simulink model "ee_converter_dcdc_llc"  (R2019b)
settings: Solver=VariableStepAuto  StartTime=0.0  StopTime=2e-3  RelTol=1e-3  AbsTol=1e-3  EnableMultiTasking=on
PreLoadFcn:
  | Vbus_nominal = 450;
  | Vbus_ripple = 10;
  | busRippleFrequency = 100;
  | Vout_nominal = 54;
  | Pout = 100;
  | Cr = 1.5e-8;
  | Lr = 2e-4;
  | Lm_theory = 2.5e-3;
  | n = 4.3;
  | transformerCoupling = 0.99;
  | Cout = 3e-5;
  | tdead = 3e-7;
  | fswfinal = [68.7 93.7]*1e3;
  | Vf = 0.6;
  | 
  | switchType = 1;
StopFcn:
  | ee_addSimlogTimeStamp(bdroot)
undefined symbols (not defined in the file or in its folder): diff
libraries: ee_lib x12, fl_lib x10, nesl_utility x6, simulink x4
(part 1 of 2)
CloseFcn:
  | try,close(h1_ee_converter_dcdc_llc),end
  | clear h1_ee_converter_dcdc_llc
  | try,close(h2_ee_converter_dcdc_llc),end
  | clear h2_ee_converter_dcdc_llc
  | try,close(h3_ee_converter_dcdc_llc),end
  | clear h3_ee_converter_dcdc_llc
  | try,close(h4_ee_converter_dcdc_llc),end
  | clear h4_ee_converter_dcdc_llc
  | try,close(h5_ee_converter_dcdc_llc),end
  | clear h5_ee_converter_dcdc_llc
  | 
  | clear simlog_ee_converter_dcdc_llc
  | clear logsout_ee_converter_dcdc_llc
  | clear simlogs_ee_converter_dcdc_llc
  | clear logsouts_ee_converter_dcdc_llc
  | 
  | clear Cout Cr G Gmax Gmax_factor Gmin Gnom Gnorm Gplot Iout Lm Lm_theory Lr Lr_theory Pout Q Qmaxfinal Qminfinal Qnomfinal Qplot Qrange Re Remax Remin Renom Vbus Vbus_nominal Vbus_ripple Vf Vout Vout_nominal Vout_ripple Zr busRippleFrequency ff ffinal fn fplot frange fsw fswfinal ii io lambda leg minLoad n nexact numCurves numPts qq showplots simlog_fctrl switchType tdead temp_ivar temp_variant tout transformerCoupling vi vo
Description:
  | DC-DC LLC Converter
settings Model: Creator=The MathWorks, Inc.  LastModifiedBy=sheldon
settings SolverCC: AutoScaleAbsTol=off  MaxConsecutiveMinStep=5
settings DataIOCC: LimitDataPoints=on  MaxDataPoints=400000  ReturnWorkspaceOutputs=off  SignalLoggingName=logsout_ee_converter_dcdc_llc
settings DebuggingCC: ArithmeticOperatorsInVariantConditions=warning
settings SFSimCC: SimUseLocalCustomCode=off  CustomCodeUndefinedFunction=UseInterfaceOnly
settings RTWCC: RTWUseLocalCustomCode=off
settings CodeAppCC: StateflowObjectComments=on
settings GRTTargetCC: TargetLangStandard=C89/C90 (ANSI)
settings ConfigComp: CovMetricSettings=dw  CovHtmlReporting=on  CovSaveCumulativeToWorkspaceVar=on  CovSaveSingleToWorkspaceVar=on  CovShowResultsExplorer=off  CovExternalEMLEnable=off
settings SimscapeCC: SimscapeLogType=all  SimscapeLogSimulationStatistics=on  SimscapeLogName=simlog_ee_converter_dcdc_llc  SimscapeLogDataHistory=400000

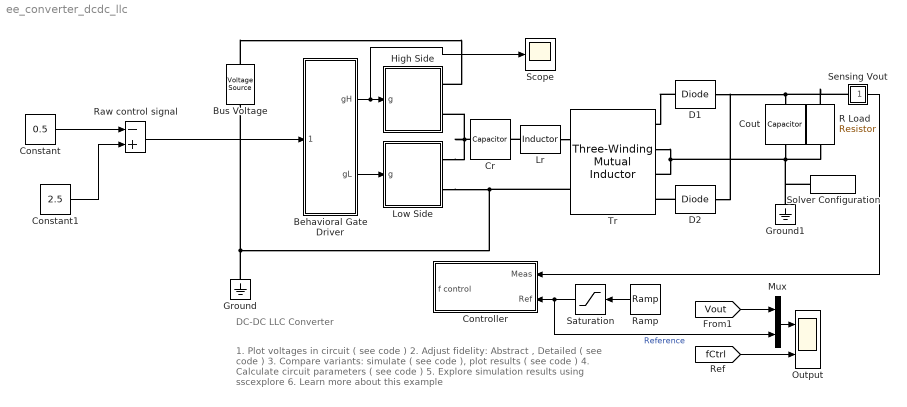
== system ee_converter_dcdc_llc ==
  note: DC-DC LLC Converter
  note: 1. Plot voltages in circuit ( see code )
      | 2. Adjust fidelity: Abstract , Detailed ( see code )
      | 3. Compare variants: simulate ( see code ), plot results ( see code )
      | 4. Calculate circuit parameters ( see code )
      | 5. Explore simulation results using sscexplore
      | 6. Learn more about this example
  Behavioral Gate Driver : Subsystem
  Bus Voltage : ee_lib/Sources/Voltage Source  dc_voltage=Vbus_nominal V  ac_voltage=Vbus_ripple V  ac_shift=0 deg  ac_frequency=busRippleFrequency Hz  noise_mode=0  PSD=0 V^2/Hz  repeatability=1  auto_seed=3499211588  user_seed=0  sample_time=0.001 s  i_specify=off  i_priority=None  i=0 A  i_nominal_specify=off  i_nominal_unit=A  i_nominal_value=1  v_specify=off  v_priority=None  v=0 V  v_nominal_specify=off  v_nominal_unit=V  v_nominal_value=1
      settings: SourceProductName=Simscape Electrical
  Constant : Constant  Value=0.5
  Constant1 : Constant  Value=2.5
  Controller : Subsystem
  Cout : ee_lib/Passive/Capacitor  cap_option=0  c=Cout F  Cvec=[ 1e-5 1e-6 ] F  Vvec=[ 0 10 ] V  CV_table_symmetry=1  f_vec=[1, 10] kHz  DFext_vec=[.8, 1.2]  C_tol=5  enable_C_tol=0  tol_distribution=1  nSigma=4  r=1e-6 Ohm  g=0 1/Ohm  averaging_period=0 s  enable_operating_limits=0  operating_limit_action=2  max_working_voltage_range=[ -25 25 ] V  power_rating=1 W  enable_faults=0  fault_action=1  Cscale_faulted=100  R_faulted=0.001 Ohm  G_faulted=0 1/Ohm  tau_fault=0.001 s  enable_temporal_fault=0  t_fault=1 s  enable_behavioral_fault=0  max_permissible_voltage_range=[ -100 100 ] V  t_fail_on_voltage=1 s  i_specify=off  i_priority=None  i=0 A  i_nominal_specify=off  i_nominal_unit=A  i_nominal_value=1  v_specify=off  v_priority=None  v=0 V  v_nominal_specify=off  v_nominal_unit=V  v_nominal_value=1  vc_specify=on  vc_priority=High  vc=0 V  vc_nominal_specify=off  vc_nominal_unit=V  vc_nominal_value=1
      settings: SourceProductName=Simscape Electrical
  Cr : ee_lib/Passive/Capacitor  cap_option=0  c=Cr F  Cvec=[ 1e-5 1e-6 ] F  Vvec=[ 0 10 ] V  CV_table_symmetry=1  f_vec=[1, 10] kHz  DFext_vec=[.8, 1.2]  C_tol=5  enable_C_tol=0  tol_distribution=1  nSigma=4  r=1e-6 Ohm  g=1e-6 1/Ohm  averaging_period=0 s  enable_operating_limits=0  operating_limit_action=2  max_working_voltage_range=[ -25 25 ] V  power_rating=1 W  enable_faults=0  fault_action=1  Cscale_faulted=100  R_faulted=0.001 Ohm  G_faulted=0 1/Ohm  tau_fault=0.001 s  enable_temporal_fault=0  t_fault=1 s  enable_behavioral_fault=0  max_permissible_voltage_range=[ -100 100 ] V  t_fail_on_voltage=1 s  i_specify=off  i_priority=None  i=0 A  i_nominal_specify=off  i_nominal_unit=A  i_nominal_value=1  v_specify=off  v_priority=None  v=0 V  v_nominal_specify=off  v_nominal_unit=V  v_nominal_value=1  vc_specify=on  vc_priority=High  vc=0 V  vc_nominal_specify=off  vc_nominal_unit=V  vc_nominal_value=1
      settings: SourceProductName=Simscape Electrical
  D1 : ee_lib/Semiconductors & Converters/Diode  ModelType=ee.enum.diode.modelType.pwl  Vf=Vf V  Ron=0.3 Ohm  Goff=1e-8 S  prmExp=1  I12=[ 0.0137 0.545 ] A  V12=[ 0.6 0.7 ] V  IS=1e-12 A  ec=1  I1=0.0137 A  V1=0.6 V  RS=0.01 Ohm  Tmeas=25 degC  N_series=1  N_parallel=1  Rz=0.3 Ohm  BV=inf V  C_param=1  CJ=0 pF  CJ0=5 pF  VJ=1 V  Mgrad=0.5  Vvec=[ 0.1 10 100 ] V  Cvec=[ 3.5 1 0.4 ] pF  FC=0.5  Q_param=ee.enum.diode.recoveryParam.off  iRM=-7.15 A  iF=4 A  didt=-750 A/us  trr_factor=3  trr=115 ns  Qrr=1500 s*uA  TT=50 ns  tau=100 ns  T_param=1  IS_T2=1.25e-7 A  I1_T2=0.245 A  V1_T2=0.5 V  Tmeas2=125 degC  EG_param=1  EG=1.11 eV  XTI_param=1  XTI=3  dBVdT=0 V/K  Tdevice=25 degC  i_specify=off  i_priority=None  i=0 A  i_nominal_specify=off  i_nominal_unit=A  i_nominal_value=1  v_specify=off  v_priority=None  v=0 V  v_nominal_specify=off  v_nominal_unit=V  v_nominal_value=1  i_capacitor_specify=off  i_capacitor_priority=High  i_capacitor=0 A  i_capacitor_nominal_specify=off  i_capacitor_nominal_unit=A  i_capacitor_nominal_value=1  v_capacitor_specify=off  v_capacitor_priority=None  v_capacitor=0 V  v_capacitor_nominal_specify=off  v_capacitor_nominal_unit=V  v_capacitor_nominal_value=1  power_dissipated_specify=off  power_dissipated_priority=None  power_dissipated=0 W  power_dissipated_nominal_specify=off  power_dissipated_nominal_unit=W  power_dissipated_nominal_value=1  thermal_network_parameterization=ee.enum.thermalNetworkTopology.cauer  Rth=[0, 10] K/W  Rth_Foster=[4, 6] K/W  thermal_mass_parameterization=ee.enum.thermalNetwork.timeconstant  thermal_mass=[0, 1] J/K  thermal_mass_Foster=[1.5, 3] J/K  thermal_time_constant=[0, 10] s  thermal_time_constant_Foster=[6, 18] s  thermal_mass_initial_temperatures=[25, 25] degC
      settings: SourceProductName=Simscape Electrical
  D2 : ee_lib/Semiconductors & Converters/Diode  ModelType=ee.enum.diode.modelType.pwl  Vf=Vf V  Ron=0.3 Ohm  Goff=1e-8 S  prmExp=1  I12=[ 0.0137 0.545 ] A  V12=[ 0.6 0.7 ] V  IS=1e-12 A  ec=1  I1=0.0137 A  V1=0.6 V  RS=0.01 Ohm  Tmeas=25 degC  N_series=1  N_parallel=1  Rz=0.3 Ohm  BV=inf V  C_param=1  CJ=0 pF  CJ0=5 pF  VJ=1 V  Mgrad=0.5  Vvec=[ 0.1 10 100 ] V  Cvec=[ 3.5 1 0.4 ] pF  FC=0.5  Q_param=ee.enum.diode.recoveryParam.off  iRM=-7.15 A  iF=4 A  didt=-750 A/us  trr_factor=3  trr=115 ns  Qrr=1500 s*uA  TT=50 ns  tau=100 ns  T_param=1  IS_T2=1.25e-7 A  I1_T2=0.245 A  V1_T2=0.5 V  Tmeas2=125 degC  EG_param=1  EG=1.11 eV  XTI_param=1  XTI=3  dBVdT=0 V/K  Tdevice=25 degC  i_specify=off  i_priority=None  i=0 A  i_nominal_specify=off  i_nominal_unit=A  i_nominal_value=1  v_specify=off  v_priority=None  v=0 V  v_nominal_specify=off  v_nominal_unit=V  v_nominal_value=1  i_capacitor_specify=off  i_capacitor_priority=High  i_capacitor=0 A  i_capacitor_nominal_specify=off  i_capacitor_nominal_unit=A  i_capacitor_nominal_value=1  v_capacitor_specify=off  v_capacitor_priority=None  v_capacitor=0 V  v_capacitor_nominal_specify=off  v_capacitor_nominal_unit=V  v_capacitor_nominal_value=1  power_dissipated_specify=off  power_dissipated_priority=None  power_dissipated=0 W  power_dissipated_nominal_specify=off  power_dissipated_nominal_unit=W  power_dissipated_nominal_value=1  thermal_network_parameterization=ee.enum.thermalNetworkTopology.cauer  Rth=[0, 10] K/W  Rth_Foster=[4, 6] K/W  thermal_mass_parameterization=ee.enum.thermalNetwork.timeconstant  thermal_mass=[0, 1] J/K  thermal_mass_Foster=[1.5, 3] J/K  thermal_time_constant=[0, 10] s  thermal_time_constant_Foster=[6, 18] s  thermal_mass_initial_temperatures=[25, 25] degC
      settings: SourceProductName=Simscape Electrical
  Ground : fl_lib/Electrical/Electrical Elements/Electrical Reference
  Ground1 : fl_lib/Electrical/Electrical Elements/Electrical Reference
  High Side : Subsystem  Variant=on
      mask Display:
      | blk = find_system(gcbh, 'SearchDepth', 1, 'Parent', gcb, 'VariantObject', get_param(gcb,'activevariant'));
      | eval(get_param(blk, 'MaskDisplay'));
  Low Side : Subsystem  Variant=on
      mask Display:
      | blk = find_system(gcbh, 'SearchDepth', 1, 'Parent', gcb, 'VariantObject', get_param(gcb,'activevariant'));
      | eval(get_param(blk, 'MaskDisplay'));
  Lr : ee_lib/Passive/Inductor  l=Lr H  L_tol=20  enable_L_tol=0  tol_distribution=1  nSigma=4  r=0 Ohm  g=1e-9 1/Ohm  enable_operating_limits=0  operating_limit_action=2  max_working_current=1 A  power_rating=1 W  enable_faults=0  fault_action=1  lambdaPercent=50  k_faulted=0.9999  turnsShort=0  openCct=0  groundShort=0  groundShortG=0 1/Ohm  tau_fault=0.001 s  enable_temporal_fault=0  t_fault=1 s  enable_behavioral_fault=0  max_permissible_voltage=100 V  n_fail_on_voltage=1  max_permissible_current=1 A  t_fail_on_current=1 s  i_L_specify=on  i_L_priority=High  i_L=0 A  i_L_nominal_specify=off  i_L_nominal_unit=A  i_L_nominal_value=1
      settings: SourceProductName=Simscape Electrical
  Mux : Mux  Inputs=2
  Output : Scope  NumInputPorts=2
  R Load : ee_lib/Passive/Resistor  R=Vout_nominal^2/Pout Ohm  R_tol=5  enable_R_tol=0  tol_distribution=1  nSigma=4  enable_operating_limits=0  operating_limit_action=2  max_working_voltage=100 V  power_rating=1 W  enable_faults=0  fault_action=1  R_faulted=Inf Ohm  enable_temporal_fault=0  t_fault=1 s  enable_behavioral_fault=0  max_permissible_current=1 A  t_fail_on_current=1 s  noise_mode=0  sample_time=0.001 s  repeatability=1  auto_seed=2241481901  user_seed=0  Tdevice=25 degC  alpha=3.93e-3 1/K  Tmeas=25 degC  thermal_mass=100 J/K  power_derating_T1=70 degC  power_derating_T2=155 degC  operating_temperature_range_vec=[-50, 150] degC  temperature_specify=off  temperature_priority=High  temperature=298.15 K  temperature_nominal_specify=off  temperature_nominal_unit=K  temperature_nominal_value=1
      settings: SourceProductName=Simscape Electrical
  Ramp : simulink/Sources/Ramp  slope=Vout_nominal/1e-3  start=0  InitialOutput=0
  Raw control signal : Sum  Inputs=-+
  Saturation : Saturate  UpperLimit=Vout_nominal  LowerLimit=0
  Scope : Scope
  Sensing Vout : Subsystem
      mask Display: disp('v')
  Solver Configuration : nesl_utility/Solver Configuration  PhysicalDomain=network_engine_domain  SubClassName=solver  LeftPortType=input  RightPortType=generic  Tones=[]  Harmonics=[]  SimulateNoise=off  Profile=off  UseLocalSampling=off  EnableSwitchedLinearOptims=on  FrequencyDomain=off  UseCCode=off  RelTol=0.001  AbsTol=1e-06  MinStep=1e-09  ToWorkspace=off  RevertToSquareIcSolve=off  NumHomotopyIterations=100  PhasorMode=off  PhasorModeNumHarmonics=1  DoDC=off  ResidualTolerance=1e-09  UseLocalSolver=off  LocalSolverChoice=NE_BACKWARD_EULER_ADVANCER  LocalSolverSampleTime=0.001  DoFixedCost=off  MaxNonlinIter=3  MaxModeIter=2  LinearAlgebra=auto  EquationFormulation=NE_TIME_EF  DelaysMemoryBudget=1024  AutomaticFiltering=on  FilteringTimeConstant=0.001  PartitionStorageMethod=AS_NEEDED  PartitionMemoryBudget=1024  PartitionMethod=FAST
  Tr : ee_lib/Passive/Transformers/Three-Winding Mutual Inductor  L1=Lm_theory H  L2=Lm_theory/n^2 H  L3=Lm_theory/n^2 H  K12=transformerCoupling  K13=transformerCoupling  K23=transformerCoupling  IC_given=1  IC1=0 A  IC2=0 A  IC3=0 A
      settings: SourceProductName=Simscape Electrical  SourceProductBaseCode=PS  InternalSimscapePortConfiguration="{\"Bottom\":[],\"Left\":[{\"id\":\"p1\",\"label\":\"1+\",\"type\":\"foundation.electrical.electrical\"},{\"id\":\"n1\",\"label\":\"1-\",\"type\":\"foundation.electrical.electrical\"}],\"Right\":[{\"id\":\"p2\",\"label\":\"2+\",\"type\":\"foundation.electrical.electrical\"},{\"id\":\"n2\",\"label\":\"2-\",\"type\":\"foundation.electrical.electrical\"},{\"id\":\"p3\",\"label\":\"3+\",\"type\":\"foundation.electrical.electrical\"},{\"id\":\"n3\",\"label\":\"3-\",\"type\":\"foundation.electrical.electrical\"}],\"Top\":[]}"
  wires:
  Behavioral Gate Driver/1(gH) -> Scope/1, High Side/1(g)
  Behavioral Gate Driver/2(gL) -> Low Side/1(g)
  Sensing Vout/1(v) -> Controller/1(Meas)
  [Vout] -> Mux/1
  Ramp/1 -> Saturation/1
  Mux/1 -> Output/1
  [fCtrl] -> Output/2
  Saturation/1 -> Mux/2, Controller/2(Ref)  "Reference"
  Constant/1 -> Raw control signal/1
  Constant1/1 -> Raw control signal/2
  Raw control signal/1 -> Behavioral Gate Driver/1(Control)
  connections:
  Lr/LConn1 -- Cr/RConn1
  Tr/RConn2 -- Tr/RConn3 -- R Load/RConn1 -- Ground1/LConn1 -- Solver Configuration/RConn1 -- Cout/RConn1
  Cr/LConn1 -- High Side/RConn2 -- Low Side/RConn1
  Ground/LConn1 -- Low Side/RConn2 -- Tr/LConn2 -- Bus Voltage/RConn1
  Lr/RConn1 -- Tr/LConn1
  Sensing Vout/LConn1 -- R Load/LConn1 -- D2/RConn1 -- D1/RConn1 -- Cout/LConn1
  D1/LConn1 -- Tr/RConn1
  D2/LConn1 -- Tr/RConn4
  Bus Voltage/LConn1 -- High Side/RConn1

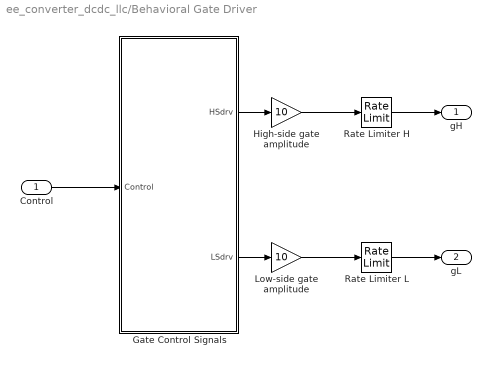
== system ee_converter_dcdc_llc/Behavioral Gate Driver ==
  Control : Inport
  Gate Control Signals : Subsystem  mask{tdead=tdead, fnom=mean(fswfinal), vnom=2.5, dfdv=diff(fswfinal)/2}
      mask prompts: tdead "Dead time"; fnom "Nominal oscillation frequency"; vnom "Nominal control value"; dfdv "Sensitivity of frequency to control value"
      mask DialogControl DescTextVar Prompt: Produces half-bridge gate control signals with a dead-time to prevent cross-conduction. The switching frequency is determined by the input control signal.
  High-side gate amplitude : Gain  Gain=10
  Low-side gate amplitude : Gain  Gain=10
  Rate Limiter H : RateLimiter  RisingSlewLimit=10*5/tdead  FallingSlewLimit=-10*5/tdead
  Rate Limiter L : RateLimiter  RisingSlewLimit=10*5/tdead  FallingSlewLimit=-10*5/tdead
  gH : Outport  VectorParamsAs1DForOutWhenUnconnected=off
  gL : Outport  Port=2  VectorParamsAs1DForOutWhenUnconnected=off
  wires:
  Control/1 -> Gate Control Signals/1(Control)
  Gate Control Signals/1(HSdrv) -> High-side gate amplitude/1
  Gate Control Signals/2(LSdrv) -> Low-side gate amplitude/1
  High-side gate amplitude/1 -> Rate Limiter H/1
  Low-side gate amplitude/1 -> Rate Limiter L/1
  Rate Limiter H/1 -> gH/1
  Rate Limiter L/1 -> gL/1

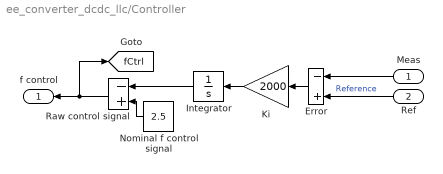
== system ee_converter_dcdc_llc/Controller ==
  Meas : Inport
  Ref : Inport  Port=2
  Error : Sum  Inputs=-+
  Integrator : Integrator  LimitOutput=on  UpperSaturationLimit=2.5  LowerSaturationLimit=-7.5
  Ki : Gain  Gain=2000
  Nominal f control signal : Constant  Value=2.5
  Raw control signal : Sum  Inputs=-+
  f control : Outport  VectorParamsAs1DForOutWhenUnconnected=off
  tag scope: fCtrl=global
  wires:
  Nominal f control signal/1 -> Raw control signal/2
  Meas/1 -> Error/1
  Ref/1 -> Error/2  "Reference"
  Ki/1 -> Integrator/1
  Error/1 -> Ki/1
  Integrator/1 -> Raw control signal/1
  Raw control signal/1 -> f control/1, [fCtrl]

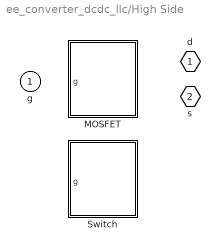
== system ee_converter_dcdc_llc/High Side ==
  g : Inport
  MOSFET : Subsystem  Tag=PublishSubsystem  VariantControl=switchType ==1
      mask Display:
      | patch([96+30;0-30;0-30;96+30], [0+20;0+20;227-20;227-20], [1;1;1])
      | plot([96.6109160799533;96.4198282107139;95.8484048836359;94.9021492177306;93.5901741723367;91.9251147843401;89.9230064858609;87.6031306742773;84.9878290218281;82.1022883130956;78.9742978825019;75.6339819878271;72.1135096971394;68.4467850830839;64.6691207081296;60.8168975452888;56.927214609459;53.0375316736292;49.1853085107884;45.4076441358342;41.7409195217787;38.220447231091;34.8801313364162;31.7521409058224;28.86660019709;26.2512985446407;23.9314227330572;21.929314434578;20.2642550465813;18.9522800011875;18.0060243352822;17.4346010082041;17.2435131389648;17.4346010082041;18.0060243352822;18.9522800011875;20.2642550465814;21.9293144345781;23.9314227330573;26.2512985446408;28.8666001970901;31.7521409058226;34.8801313364163;38.2204472310911;41.7409195217788;45.4076441358342;49.1853085107884;53.0375316736292;56.927214609459;60.8168975452889;64.6691207081297;68.4467850830839;72.1135096971393;75.633981987827;78.9742978825018;82.1022883130955;84.9878290218281;87.6031306742773;89.9230064858608;91.9251147843399;93.5901741723367;94.9021492177305;95.8484048836358;96.4198282107139;96.6109160799533;96.6109160799533], [113.618216710165;109.728533774335;105.876310611494;102.09864623654;98.4319216224848;94.9114493317971;91.5711334371223;88.4431430065286;85.5576022977961;82.9423006453468;80.6224248337633;78.6203165352841;76.9552571472875;75.6432821018936;74.6970264359883;74.1256031089102;73.9345152396709;74.1256031089102;74.6970264359883;75.6432821018936;76.9552571472875;78.6203165352842;80.6224248337634;82.9423006453469;85.5576022977961;88.4431430065287;91.5711334371223;94.9114493317971;98.4319216224849;102.09864623654;105.876310611495;109.728533774335;113.618216710165;117.507899645995;121.360122808836;125.13778718379;128.804511797846;132.324984088533;135.665299983208;138.793290413802;141.678831122534;144.294132774983;146.614008586567;148.616116885046;150.281176273043;151.593151318437;152.539406984342;153.11083031142;153.301918180659;153.11083031142;152.539406984342;151.593151318437;150.281176273043;148.616116885046;146.614008586567;144.294132774983;141.678831122534;138.793290413802;135.665299983208;132.324984088533;128.804511797846;125.13778718379;121.360122808836;117.507899645995;113.618216710165;113.618216710165])
      | plot([33.9988537598401;34.5027737785131], [113.618216710165;113.618216710165])
      | plot([0.236212508752942;34.2508137691766], [113.618216710165;113.618216710165])
      | plot([34.2508137691766;34.2508137691766], [136.294617550448;90.9418158698827])
      | plot([45.5890141893178;45.5890141893178], [136.294617550448;90.9418158698827])
      | plot([45.5890141893178;68.2654150296003], [130.625517340377;130.625517340377])
      | plot([68.2654150296003;68.2654150296003], [130.625517340377;170.309218810871])
      | plot([68.2654150296003;93.776365974918], [170.309218810871;170.309218810871])
      | plot([45.5890141893178;68.2654150296003], [96.6109160799533;96.6109160799533])
      | plot([68.2654150296003;68.2654150296003], [96.6109160799533;56.927214609459])
      | plot([68.2654150296003;96.6109160799533], [56.927214609459;56.927214609459])
      | plot([45.5890141893178;68.2654150296003], [113.618216710165;113.618216710165])
      | plot([68.2654150296003;68.2654150296003], [130.618216710165;113.6109160799533])
      | plot([62.2581143993884;51.5963148195297;62.2581143993884;], [124.956417130306;113.618216710165;102.280016290024])
  Switch : Subsystem  Tag=PublishSubsystem  VariantControl=switchType ==2
      mask Display:
      | patch([113.618216710165;112.834106023101;112.057546750592;111.296017582942;110.556852462331;109.847169952939;109.173804685282;108.543241534988;107.961553169894;107.43434156694;106.966684062065;106.563084452689;106.22742962368;105.962952114529;105.772198988228;105.657007301658;105.618486413732;105.657007301658;105.772198988228;105.962952114529;106.22742962368;106.563084452689;106.966684062065;107.43434156694;107.961553169894;108.543241534988;109.173804685282;109.847169952939;110.556852462331;111.296017582942;112.057546750592;112.834106023101;113.618216710165;114.402327397229;115.178886669738;115.940415837388;116.679580957999;117.389263467392;118.062628735048;118.693191885343;119.274880250436;119.80209185339;120.269749358265;120.673348967641;121.00900379665;121.273481305801;121.464234432102;121.579426118672;121.617947006598;121.579426118672;121.464234432102;121.273481305801;121.00900379665;120.673348967641;120.269749358265;119.80209185339;119.274880250436;118.693191885343;118.062628735048;117.389263467392;116.679580957999;115.940415837388;115.178886669738;114.402327397229;113.618216710165;113.618216710165], [178.308949107304;178.270428219378;178.155236532808;177.964483406507;177.700005897356;177.364351068347;176.960751458971;176.493093954097;175.965882351142;175.384193986049;174.753630835755;174.080265568098;173.370583058705;172.631417938094;171.869888770445;171.093329497935;170.309218810871;169.525108123807;168.748548851298;167.987019683648;167.247854563037;166.538172053645;165.864806785988;165.234243635694;164.6525552706;164.125343667646;163.657686162771;163.254086553395;162.918431724386;162.653954215236;162.463201088934;162.348009402364;162.309488514438;162.348009402364;162.463201088934;162.653954215236;162.918431724386;163.254086553395;163.657686162771;164.125343667646;164.6525552706;165.234243635694;165.864806785988;166.538172053645;167.247854563037;167.987019683648;168.748548851298;169.525108123807;170.309218810871;171.093329497935;171.869888770445;172.631417938094;173.370583058705;174.080265568098;174.753630835754;175.384193986049;175.965882351142;176.493093954096;176.960751458971;177.364351068347;177.700005897356;177.964483406507;178.155236532808;178.270428219378;178.308949107304;178.308949107304], [0;0;0])
      | plot([113.618216710165;112.834106023101;112.057546750592;111.296017582942;110.556852462331;109.847169952939;109.173804685282;108.543241534988;107.961553169894;107.43434156694;106.966684062065;106.563084452689;106.22742962368;105.962952114529;105.772198988228;105.657007301658;105.618486413732;105.657007301658;105.772198988228;105.962952114529;106.22742962368;106.563084452689;106.966684062065;107.43434156694;107.961553169894;108.543241534988;109.173804685282;109.847169952939;110.556852462331;111.296017582942;112.057546750592;112.834106023101;113.618216710165;114.402327397229;115.178886669738;115.940415837388;116.679580957999;117.389263467392;118.062628735048;118.693191885343;119.274880250436;119.80209185339;120.269749358265;120.673348967641;121.00900379665;121.273481305801;121.464234432102;121.579426118672;121.617947006598;121.579426118672;121.464234432102;121.273481305801;121.00900379665;120.673348967641;120.269749358265;119.80209185339;119.274880250436;118.693191885343;118.062628735048;117.389263467392;116.679580957999;115.940415837388;115.178886669738;114.402327397229;113.618216710165;113.618216710165],[178.308949107304;178.270428219378;178.155236532808;177.964483406507;177.700005897356;177.364351068347;176.960751458971;176.493093954097;175.965882351142;175.384193986049;174.753630835755;174.080265568098;173.370583058705;172.631417938094;171.869888770445;171.093329497935;170.309218810871;169.525108123807;168.748548851298;167.987019683648;167.247854563037;166.538172053645;165.864806785988;165.234243635694;164.6525552706;164.125343667646;163.657686162771;163.254086553395;162.918431724386;162.653954215236;162.463201088934;162.348009402364;162.309488514438;162.348009402364;162.463201088934;162.653954215236;162.918431724386;163.254086553395;163.657686162771;164.125343667646;164.6525552706;165.234243635694;165.864806785988;166.538172053645;167.247854563037;167.987019683648;168.748548851298;169.525108123807;170.309218810871;171.093329497935;171.869888770445;172.631417938094;173.370583058705;174.080265568098;174.753630835754;175.384193986049;175.965882351142;176.493093954096;176.960751458971;177.364351068347;177.700005897356;177.964483406507;178.155236532808;178.270428219378;178.308949107304;178.308949107304])
      | patch([113.618216710165;112.834106023101;112.057546750592;111.296017582942;110.556852462331;109.847169952939;109.173804685282;108.543241534988;107.961553169894;107.43434156694;106.966684062065;106.563084452689;106.22742962368;105.962952114529;105.772198988228;105.657007301658;105.618486413732;105.657007301658;105.772198988228;105.962952114529;106.22742962368;106.563084452689;106.966684062065;107.43434156694;107.961553169894;108.543241534988;109.173804685282;109.847169952939;110.556852462331;111.296017582942;112.057546750592;112.834106023101;113.618216710165;114.402327397229;115.178886669738;115.940415837388;116.679580957999;117.389263467392;118.062628735048;118.693191885343;119.274880250436;119.80209185339;120.269749358265;120.673348967641;121.00900379665;121.273481305801;121.464234432102;121.579426118672;121.617947006598;121.579426118672;121.464234432102;121.273481305801;121.00900379665;120.673348967641;120.269749358265;119.80209185339;119.274880250436;118.693191885343;118.062628735048;117.389263467392;116.679580957999;115.940415837388;115.178886669738;114.402327397229;113.618216710165;113.618216710165], [64.926944905892;64.888424017966;64.7732323313963;64.5824792050947;64.3180016959439;63.9823468669351;63.5787472575591;63.1110897526843;62.5838781497303;62.0021897846366;61.3716266343423;60.6982613666856;59.988578857293;59.2494137366818;58.4878845690323;57.7113252965232;56.927214609459;56.1431039223949;55.3665446498857;54.6050154822362;53.8658503616251;53.1561678522324;52.4828025845758;51.8522394342815;51.2705510691878;50.7433394662337;50.275681961359;49.872082351983;49.5364275229742;49.2719500138234;49.0811968875218;48.9660052009521;48.9274843130261;48.9660052009521;49.0811968875218;49.2719500138234;49.5364275229742;49.8720823519831;50.275681961359;50.7433394662338;51.2705510691878;51.8522394342816;52.4828025845758;53.1561678522325;53.8658503616251;54.6050154822362;55.3665446498858;56.143103922395;56.927214609459;57.7113252965232;58.4878845690323;59.2494137366818;59.988578857293;60.6982613666856;61.3716266343422;62.0021897846366;62.5838781497303;63.1110897526843;63.5787472575591;63.982346866935;64.3180016959439;64.5824792050947;64.7732323313963;64.888424017966;64.926944905892;64.926944905892], [0;0;0])
      | plot([113.618216710165;112.834106023101;112.057546750592;111.296017582942;110.556852462331;109.847169952939;109.173804685282;108.543241534988;107.961553169894;107.43434156694;106.966684062065;106.563084452689;106.22742962368;105.962952114529;105.772198988228;105.657007301658;105.618486413732;105.657007301658;105.772198988228;105.962952114529;106.22742962368;106.563084452689;106.966684062065;107.43434156694;107.961553169894;108.543241534988;109.173804685282;109.847169952939;110.556852462331;111.296017582942;112.057546750592;112.834106023101;113.618216710165;114.402327397229;115.178886669738;115.940415837388;116.679580957999;117.389263467392;118.062628735048;118.693191885343;119.274880250436;119.80209185339;120.269749358265;120.673348967641;121.00900379665;121.273481305801;121.464234432102;121.579426118672;121.617947006598;121.579426118672;121.464234432102;121.273481305801;121.00900379665;120.673348967641;120.269749358265;119.80209185339;119.274880250436;118.693191885343;118.062628735048;117.389263467392;116.679580957999;115.940415837388;115.178886669738;114.402327397229;113.618216710165;113.618216710165], [64.926944905892;64.888424017966;64.7732323313963;64.5824792050947;64.3180016959439;63.9823468669351;63.5787472575591;63.1110897526843;62.5838781497303;62.0021897846366;61.3716266343423;60.6982613666856;59.988578857293;59.2494137366818;58.4878845690323;57.7113252965232;56.927214609459;56.1431039223949;55.3665446498857;54.6050154822362;53.8658503616251;53.1561678522324;52.4828025845758;51.8522394342815;51.2705510691878;50.7433394662337;50.275681961359;49.872082351983;49.5364275229742;49.2719500138234;49.0811968875218;48.9660052009521;48.9274843130261;48.9660052009521;49.0811968875218;49.2719500138234;49.5364275229742;49.8720823519831;50.275681961359;50.7433394662338;51.2705510691878;51.8522394342816;52.4828025845758;53.1561678522325;53.8658503616251;54.6050154822362;55.3665446498858;56.143103922395;56.927214609459;57.7113252965232;58.4878845690323;59.2494137366818;59.988578857293;60.6982613666856;61.3716266343422;62.0021897846366;62.5838781497303;63.1110897526843;63.5787472575591;63.982346866935;64.3180016959439;64.5824792050947;64.7732323313963;64.888424017966;64.926944905892;64.926944905892])
      | plot([113.618216710165;56.927214609459], [56.927214609459;161.805568495765])
      | patch([227.23643342033;227.23643342033;0;0;227.23643342033;226.764008402824;0.472425017505884;0.472425017505884;226.764008402824;226.764008402824;227.23643342033], [0;227.23643342033;227.23643342033;0;0;0.472425017505884;0.472425017505884;226.764008402824;226.764008402824;0.472425017505884;0], [1;1;1])
      | plot([113.618216710165;186.927214609459], [170.309218810871;170.309218810871])
      | plot([113.618216710165;186.927214609459], [56.927214609459;56.927214609459])
      | % Diode
      | plot([113;113]+20, [170.309218810871;56.927214609459]);
      | patch([115;115+15;115-15]+21,[130;100;100],[0;0;0]);
      | plot([130;100]+21, [130;130]);
      | 
      | % Capacitor
      | plot([113;113]+60, [170;125]);
      | plot([113;113]+60, [110;56]);
      | plot([130;100]+60, [125;125]);
      | plot([130;100]+60, [110;110]);
      | 
      | % Switch
      | plot([30 90],[105 105])
  d : PMIOPort  Side=Right
  s : PMIOPort  Port=2  Side=Right

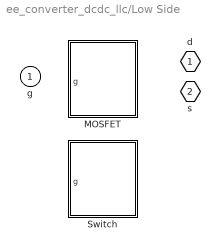
== system ee_converter_dcdc_llc/Low Side ==
  g : Inport
  MOSFET : Subsystem  VariantControl=switchType ==1
      mask Display:
      | patch([96+30;0-30;0-30;96+30], [0+20;0+20;227-20;227-20], [1;1;1])
      | plot([96.6109160799533;96.4198282107139;95.8484048836359;94.9021492177306;93.5901741723367;91.9251147843401;89.9230064858609;87.6031306742773;84.9878290218281;82.1022883130956;78.9742978825019;75.6339819878271;72.1135096971394;68.4467850830839;64.6691207081296;60.8168975452888;56.927214609459;53.0375316736292;49.1853085107884;45.4076441358342;41.7409195217787;38.220447231091;34.8801313364162;31.7521409058224;28.86660019709;26.2512985446407;23.9314227330572;21.929314434578;20.2642550465813;18.9522800011875;18.0060243352822;17.4346010082041;17.2435131389648;17.4346010082041;18.0060243352822;18.9522800011875;20.2642550465814;21.9293144345781;23.9314227330573;26.2512985446408;28.8666001970901;31.7521409058226;34.8801313364163;38.2204472310911;41.7409195217788;45.4076441358342;49.1853085107884;53.0375316736292;56.927214609459;60.8168975452889;64.6691207081297;68.4467850830839;72.1135096971393;75.633981987827;78.9742978825018;82.1022883130955;84.9878290218281;87.6031306742773;89.9230064858608;91.9251147843399;93.5901741723367;94.9021492177305;95.8484048836358;96.4198282107139;96.6109160799533;96.6109160799533], [113.618216710165;109.728533774335;105.876310611494;102.09864623654;98.4319216224848;94.9114493317971;91.5711334371223;88.4431430065286;85.5576022977961;82.9423006453468;80.6224248337633;78.6203165352841;76.9552571472875;75.6432821018936;74.6970264359883;74.1256031089102;73.9345152396709;74.1256031089102;74.6970264359883;75.6432821018936;76.9552571472875;78.6203165352842;80.6224248337634;82.9423006453469;85.5576022977961;88.4431430065287;91.5711334371223;94.9114493317971;98.4319216224849;102.09864623654;105.876310611495;109.728533774335;113.618216710165;117.507899645995;121.360122808836;125.13778718379;128.804511797846;132.324984088533;135.665299983208;138.793290413802;141.678831122534;144.294132774983;146.614008586567;148.616116885046;150.281176273043;151.593151318437;152.539406984342;153.11083031142;153.301918180659;153.11083031142;152.539406984342;151.593151318437;150.281176273043;148.616116885046;146.614008586567;144.294132774983;141.678831122534;138.793290413802;135.665299983208;132.324984088533;128.804511797846;125.13778718379;121.360122808836;117.507899645995;113.618216710165;113.618216710165])
      | plot([33.9988537598401;34.5027737785131], [113.618216710165;113.618216710165])
      | plot([0.236212508752942;34.2508137691766], [113.618216710165;113.618216710165])
      | plot([34.2508137691766;34.2508137691766], [136.294617550448;90.9418158698827])
      | plot([45.5890141893178;45.5890141893178], [136.294617550448;90.9418158698827])
      | plot([45.5890141893178;68.2654150296003], [130.625517340377;130.625517340377])
      | plot([68.2654150296003;68.2654150296003], [130.625517340377;170.309218810871])
      | plot([68.2654150296003;93.776365974918], [170.309218810871;170.309218810871])
      | plot([45.5890141893178;68.2654150296003], [96.6109160799533;96.6109160799533])
      | plot([68.2654150296003;68.2654150296003], [96.6109160799533;56.927214609459])
      | plot([68.2654150296003;96.6109160799533], [56.927214609459;56.927214609459])
      | plot([45.5890141893178;68.2654150296003], [113.618216710165;113.618216710165])
      | plot([68.2654150296003;68.2654150296003], [130.618216710165;113.6109160799533])
      | plot([62.2581143993884;51.5963148195297;62.2581143993884;], [124.956417130306;113.618216710165;102.280016290024])
  Switch : Subsystem  VariantControl=switchType ==2
      mask Display:
      | patch([113.618216710165;112.834106023101;112.057546750592;111.296017582942;110.556852462331;109.847169952939;109.173804685282;108.543241534988;107.961553169894;107.43434156694;106.966684062065;106.563084452689;106.22742962368;105.962952114529;105.772198988228;105.657007301658;105.618486413732;105.657007301658;105.772198988228;105.962952114529;106.22742962368;106.563084452689;106.966684062065;107.43434156694;107.961553169894;108.543241534988;109.173804685282;109.847169952939;110.556852462331;111.296017582942;112.057546750592;112.834106023101;113.618216710165;114.402327397229;115.178886669738;115.940415837388;116.679580957999;117.389263467392;118.062628735048;118.693191885343;119.274880250436;119.80209185339;120.269749358265;120.673348967641;121.00900379665;121.273481305801;121.464234432102;121.579426118672;121.617947006598;121.579426118672;121.464234432102;121.273481305801;121.00900379665;120.673348967641;120.269749358265;119.80209185339;119.274880250436;118.693191885343;118.062628735048;117.389263467392;116.679580957999;115.940415837388;115.178886669738;114.402327397229;113.618216710165;113.618216710165], [178.308949107304;178.270428219378;178.155236532808;177.964483406507;177.700005897356;177.364351068347;176.960751458971;176.493093954097;175.965882351142;175.384193986049;174.753630835755;174.080265568098;173.370583058705;172.631417938094;171.869888770445;171.093329497935;170.309218810871;169.525108123807;168.748548851298;167.987019683648;167.247854563037;166.538172053645;165.864806785988;165.234243635694;164.6525552706;164.125343667646;163.657686162771;163.254086553395;162.918431724386;162.653954215236;162.463201088934;162.348009402364;162.309488514438;162.348009402364;162.463201088934;162.653954215236;162.918431724386;163.254086553395;163.657686162771;164.125343667646;164.6525552706;165.234243635694;165.864806785988;166.538172053645;167.247854563037;167.987019683648;168.748548851298;169.525108123807;170.309218810871;171.093329497935;171.869888770445;172.631417938094;173.370583058705;174.080265568098;174.753630835754;175.384193986049;175.965882351142;176.493093954096;176.960751458971;177.364351068347;177.700005897356;177.964483406507;178.155236532808;178.270428219378;178.308949107304;178.308949107304], [0;0;0])
      | plot([113.618216710165;112.834106023101;112.057546750592;111.296017582942;110.556852462331;109.847169952939;109.173804685282;108.543241534988;107.961553169894;107.43434156694;106.966684062065;106.563084452689;106.22742962368;105.962952114529;105.772198988228;105.657007301658;105.618486413732;105.657007301658;105.772198988228;105.962952114529;106.22742962368;106.563084452689;106.966684062065;107.43434156694;107.961553169894;108.543241534988;109.173804685282;109.847169952939;110.556852462331;111.296017582942;112.057546750592;112.834106023101;113.618216710165;114.402327397229;115.178886669738;115.940415837388;116.679580957999;117.389263467392;118.062628735048;118.693191885343;119.274880250436;119.80209185339;120.269749358265;120.673348967641;121.00900379665;121.273481305801;121.464234432102;121.579426118672;121.617947006598;121.579426118672;121.464234432102;121.273481305801;121.00900379665;120.673348967641;120.269749358265;119.80209185339;119.274880250436;118.693191885343;118.062628735048;117.389263467392;116.679580957999;115.940415837388;115.178886669738;114.402327397229;113.618216710165;113.618216710165],[178.308949107304;178.270428219378;178.155236532808;177.964483406507;177.700005897356;177.364351068347;176.960751458971;176.493093954097;175.965882351142;175.384193986049;174.753630835755;174.080265568098;173.370583058705;172.631417938094;171.869888770445;171.093329497935;170.309218810871;169.525108123807;168.748548851298;167.987019683648;167.247854563037;166.538172053645;165.864806785988;165.234243635694;164.6525552706;164.125343667646;163.657686162771;163.254086553395;162.918431724386;162.653954215236;162.463201088934;162.348009402364;162.309488514438;162.348009402364;162.463201088934;162.653954215236;162.918431724386;163.254086553395;163.657686162771;164.125343667646;164.6525552706;165.234243635694;165.864806785988;166.538172053645;167.247854563037;167.987019683648;168.748548851298;169.525108123807;170.309218810871;171.093329497935;171.869888770445;172.631417938094;173.370583058705;174.080265568098;174.753630835754;175.384193986049;175.965882351142;176.493093954096;176.960751458971;177.364351068347;177.700005897356;177.964483406507;178.155236532808;178.270428219378;178.308949107304;178.308949107304])
      | patch([113.618216710165;112.834106023101;112.057546750592;111.296017582942;110.556852462331;109.847169952939;109.173804685282;108.543241534988;107.961553169894;107.43434156694;106.966684062065;106.563084452689;106.22742962368;105.962952114529;105.772198988228;105.657007301658;105.618486413732;105.657007301658;105.772198988228;105.962952114529;106.22742962368;106.563084452689;106.966684062065;107.43434156694;107.961553169894;108.543241534988;109.173804685282;109.847169952939;110.556852462331;111.296017582942;112.057546750592;112.834106023101;113.618216710165;114.402327397229;115.178886669738;115.940415837388;116.679580957999;117.389263467392;118.062628735048;118.693191885343;119.274880250436;119.80209185339;120.269749358265;120.673348967641;121.00900379665;121.273481305801;121.464234432102;121.579426118672;121.617947006598;121.579426118672;121.464234432102;121.273481305801;121.00900379665;120.673348967641;120.269749358265;119.80209185339;119.274880250436;118.693191885343;118.062628735048;117.389263467392;116.679580957999;115.940415837388;115.178886669738;114.402327397229;113.618216710165;113.618216710165], [64.926944905892;64.888424017966;64.7732323313963;64.5824792050947;64.3180016959439;63.9823468669351;63.5787472575591;63.1110897526843;62.5838781497303;62.0021897846366;61.3716266343423;60.6982613666856;59.988578857293;59.2494137366818;58.4878845690323;57.7113252965232;56.927214609459;56.1431039223949;55.3665446498857;54.6050154822362;53.8658503616251;53.1561678522324;52.4828025845758;51.8522394342815;51.2705510691878;50.7433394662337;50.275681961359;49.872082351983;49.5364275229742;49.2719500138234;49.0811968875218;48.9660052009521;48.9274843130261;48.9660052009521;49.0811968875218;49.2719500138234;49.5364275229742;49.8720823519831;50.275681961359;50.7433394662338;51.2705510691878;51.8522394342816;52.4828025845758;53.1561678522325;53.8658503616251;54.6050154822362;55.3665446498858;56.143103922395;56.927214609459;57.7113252965232;58.4878845690323;59.2494137366818;59.988578857293;60.6982613666856;61.3716266343422;62.0021897846366;62.5838781497303;63.1110897526843;63.5787472575591;63.982346866935;64.3180016959439;64.5824792050947;64.7732323313963;64.888424017966;64.926944905892;64.926944905892], [0;0;0])
      | plot([113.618216710165;112.834106023101;112.057546750592;111.296017582942;110.556852462331;109.847169952939;109.173804685282;108.543241534988;107.961553169894;107.43434156694;106.966684062065;106.563084452689;106.22742962368;105.962952114529;105.772198988228;105.657007301658;105.618486413732;105.657007301658;105.772198988228;105.962952114529;106.22742962368;106.563084452689;106.966684062065;107.43434156694;107.961553169894;108.543241534988;109.173804685282;109.847169952939;110.556852462331;111.296017582942;112.057546750592;112.834106023101;113.618216710165;114.402327397229;115.178886669738;115.940415837388;116.679580957999;117.389263467392;118.062628735048;118.693191885343;119.274880250436;119.80209185339;120.269749358265;120.673348967641;121.00900379665;121.273481305801;121.464234432102;121.579426118672;121.617947006598;121.579426118672;121.464234432102;121.273481305801;121.00900379665;120.673348967641;120.269749358265;119.80209185339;119.274880250436;118.693191885343;118.062628735048;117.389263467392;116.679580957999;115.940415837388;115.178886669738;114.402327397229;113.618216710165;113.618216710165], [64.926944905892;64.888424017966;64.7732323313963;64.5824792050947;64.3180016959439;63.9823468669351;63.5787472575591;63.1110897526843;62.5838781497303;62.0021897846366;61.3716266343423;60.6982613666856;59.988578857293;59.2494137366818;58.4878845690323;57.7113252965232;56.927214609459;56.1431039223949;55.3665446498857;54.6050154822362;53.8658503616251;53.1561678522324;52.4828025845758;51.8522394342815;51.2705510691878;50.7433394662337;50.275681961359;49.872082351983;49.5364275229742;49.2719500138234;49.0811968875218;48.9660052009521;48.9274843130261;48.9660052009521;49.0811968875218;49.2719500138234;49.5364275229742;49.8720823519831;50.275681961359;50.7433394662338;51.2705510691878;51.8522394342816;52.4828025845758;53.1561678522325;53.8658503616251;54.6050154822362;55.3665446498858;56.143103922395;56.927214609459;57.7113252965232;58.4878845690323;59.2494137366818;59.988578857293;60.6982613666856;61.3716266343422;62.0021897846366;62.5838781497303;63.1110897526843;63.5787472575591;63.982346866935;64.3180016959439;64.5824792050947;64.7732323313963;64.888424017966;64.926944905892;64.926944905892])
      | plot([113.618216710165;56.927214609459], [56.927214609459;161.805568495765])
      | patch([227.23643342033;227.23643342033;0;0;227.23643342033;226.764008402824;0.472425017505884;0.472425017505884;226.764008402824;226.764008402824;227.23643342033], [0;227.23643342033;227.23643342033;0;0;0.472425017505884;0.472425017505884;226.764008402824;226.764008402824;0.472425017505884;0], [1;1;1])
      | plot([113.618216710165;186.927214609459], [170.309218810871;170.309218810871])
      | plot([113.618216710165;186.927214609459], [56.927214609459;56.927214609459])
      | % Diode
      | plot([113;113]+20, [170.309218810871;56.927214609459]);
      | patch([115;115+15;115-15]+21,[130;100;100],[0;0;0]);
      | plot([130;100]+21, [130;130]);
      | 
      | % Capacitor
      | plot([113;113]+60, [170;125]);
      | plot([113;113]+60, [110;56]);
      | plot([130;100]+60, [125;125]);
      | plot([130;100]+60, [110;110]);
      | 
      | % Switch
      | plot([30 90],[105 105])
  d : PMIOPort  Side=Right
  s : PMIOPort  Port=2  Side=Right

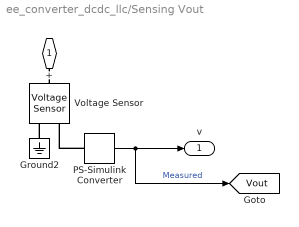
== system ee_converter_dcdc_llc/Sensing Vout ==
  Ground2 : fl_lib/Electrical/Electrical Elements/Electrical Reference
  PS-Simulink Converter : nesl_utility/PS-Simulink Converter  PhysicalDomain=network_engine_domain  SubClassName=ps_output  LeftPortType=input  RightPortType=output  PseudoPeriodic=off  Frequencies=[]  Unit=1  AffineConversion=off
  Voltage Sensor : fl_lib/Electrical/Electrical Sensors/Voltage Sensor
  + : PMIOPort  Side=Left
  v : Outport  VectorParamsAs1DForOutWhenUnconnected=off
  tag scope: Vout=global
  wires:
  PS-Simulink Converter/1 -> [Vout], v/1  "Measured"
  connections:
  PS-Simulink Converter/LConn1 -- Voltage Sensor/RConn1
  Ground2/LConn1 -- Voltage Sensor/RConn2
  Voltage Sensor/LConn1 -- +/RConn1

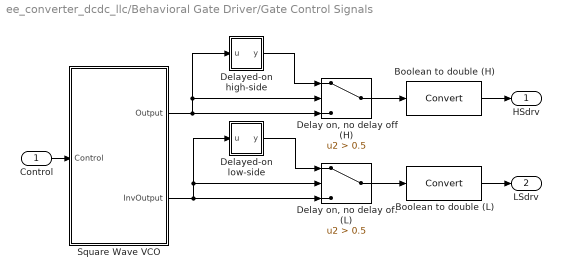
== system ee_converter_dcdc_llc/Behavioral Gate Driver/Gate Control Signals ==
  Control : Inport
  Boolean to double (H) : DataTypeConversion
  Boolean to double (L) : DataTypeConversion
  "Delay on, no delay off (H)" : Switch  Criteria=u2 > Threshold  Threshold=0.5
  "Delay on, no delay off (L)" : Switch  Criteria=u2 > Threshold  Threshold=0.5
  Delayed-on high-side : Subsystem
  "Delayed-on low-side " : Subsystem
  Square Wave VCO : Subsystem  mask{fnom=fnom, vnom=vnom, dfdv=dfdv}
      mask prompts: fnom "Nominal frequency"; vnom "Nominal control voltage"; dfdv "Rate of change of frequency with control signal"
      mask DialogControl DescTextVar Prompt: Ideal controlled oscillator. The oscillation frequency of the output depends linearly on the input signal.
  HSdrv : Outport  VectorParamsAs1DForOutWhenUnconnected=off
  LSdrv : Outport  Port=2  VectorParamsAs1DForOutWhenUnconnected=off
  wires:
  Delayed-on high-side/1(y) -> "Delay on, no delay off (H)"/1
  Square Wave VCO/2(InvOutput) -> "Delayed-on low-side "/1(u), "Delay on, no delay off (L)"/2, "Delay on, no delay off (L)"/3
  "Delayed-on low-side "/1(y) -> "Delay on, no delay off (L)"/1
  "Delay on, no delay off (H)"/1 -> Boolean to double (H)/1
  "Delay on, no delay off (L)"/1 -> Boolean to double (L)/1
  Control/1 -> Square Wave VCO/1(Control)
  Square Wave VCO/1(Output) -> Delayed-on high-side/1(u), "Delay on, no delay off (H)"/2, "Delay on, no delay off (H)"/3
  Boolean to double (H)/1 -> HSdrv/1
  Boolean to double (L)/1 -> LSdrv/1

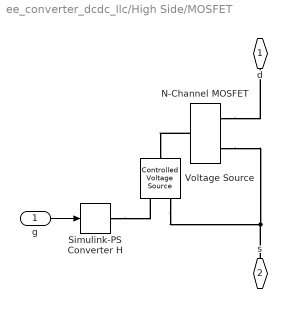
== system ee_converter_dcdc_llc/High Side/MOSFET ==
  g : Inport
  N-Channel MOSFET : ee_lib/Semiconductors & Converters/N-Channel MOSFET  parameterization=1  prmDatasheet=1  prmEquCoeff=1  Beta=5.0 A/V^2  Rds=0.025 Ohm  Id=6.0 A  Vgs=10 V  Vth=1.7 V  lam=0 1/V  Tmeas=25 degC  RS=0.0001 Ohm  RD=0.01 Ohm  C_param=1  C_GS=270 pF  C_GD=80 pF  C_DS=0 pF  C_iss=350 pF  C_rss=80 pF  C_oss=0 pF  C_GS_vec=[270, 300, 290, 280, 295, 255] pF  C_GD_vec=[450, 400, 300, 190, 95, 55] pF  C_DS_vec=[450, 410, 390, 230, 175, 115] pF  C_iss_vec=[720, 700, 590, 470, 390, 310] pF  C_rss_vec=[450, 400, 300, 190, 95, 55] pF  C_oss_vec=[900, 810, 690, 420, 270, 170] pF  C_Vds_vec=[.1, .3, 1, 3, 10, 30] V  V_GS_for_cap_data=0 V  charge_linearity_param=1  C_OX=200 pF  V_C_OX=-0.5 V  IsDiode=0 A  Vbi=1.2 V  n=1  Cj0Diode=0 pF  TT=430 ns  dVth_dT=-6 mV/K  Rds_T2=0.037 Ohm  Tmeas2=125 degC  BEXDatasheet=-1.5  BEXEquCoeff=-1.5  etaisDatasheet=3  etaisEquCoeff=3  TdeviceDatasheet=25 degC  TdeviceEquCoeff=25 degC  thermal_network_parameterization=ee.enum.thermalNetworkTopology.cauer  Rth=[0, 10] K/W  Rth_Foster=[4, 6] K/W  thermal_mass_parameterization=ee.enum.thermalNetwork.timeconstant  thermal_mass=[0, 1] J/K  thermal_mass_Foster=[1.5, 3] J/K  thermal_time_constant=[0, 10] s  thermal_time_constant_Foster=[6, 18] s  thermal_mass_initial_temperatures=[25, 25] degC  betaref=18 A/V^2  Vfbref=- 1.1 V  gamma=3.5 V^0.50000  phib2ref=1 V  thesatref=0.4 1/V  alpha=0  Vp=5e-2 V  thesrref=0 1/V  m=2  Tref=298.15 K  Cox=1500 pF  Cgso=100 pF  Cgdo=14 pF  Rsref=2e-3 Ohm  Rdref=0.17 Ohm  Rgref=8.4 Ohm  Isref=5.2e-13 A  Cj0=480 pF  Tprm=1  etabet=1.3  Stvfb=5e-4 V/K  Stphib=- 8.5e-4 V/K  etasat=1.04  etasr=0.65  etar=0.95  etais=3  Tsim=298.15 K  T0=[25, 25] degC
      settings: SourceProductName=Simscape Electrical
  Simulink-PS Converter H : nesl_utility/Simulink-PS Converter  PhysicalDomain=network_engine_domain  SubClassName=ps_input  LeftPortType=input  RightPortType=output  PseudoPeriodic=off  Frequencies=[]  NoiseDistribution=none  NoiseParameters=[]  Unit=1  AffineConversion=off  FilteringAndDerivatives=zero  SimscapeFilterOrder=1  InputFilterTimeConstant=0.001  UdotUserProvided=1
  Voltage Source : fl_lib/Electrical/Electrical Sources/Controlled Voltage Source
  d : PMIOPort  Side=Right
  s : PMIOPort  Port=2  Side=Right
  wires:
  g/1 -> Simulink-PS Converter H/1
  connections:
  N-Channel MOSFET/RConn1 -- d/RConn1
  N-Channel MOSFET/LConn1 -- Voltage Source/LConn1
  Simulink-PS Converter H/RConn1 -- Voltage Source/RConn1
  s/RConn1 -- Voltage Source/RConn2 -- N-Channel MOSFET/RConn2
